simulink model "if_else"  (R2021a)
settings: Solver=VariableStepAuto  StartTime=0.0  StopTime=inf  MaxStep=0.01  RelTol=1e-3
libraries: simulink x1
settings Model: Creator=Aula  LastModifiedBy=Aula

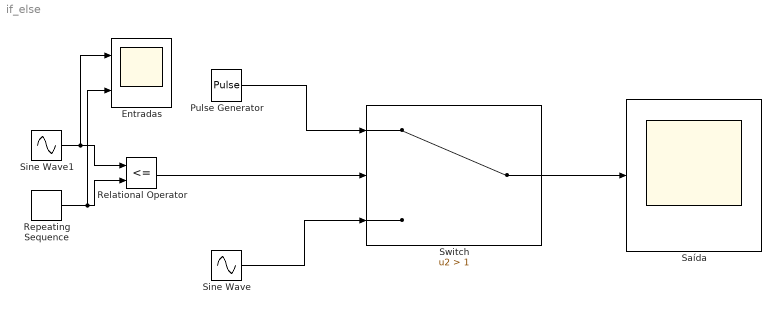
== system if_else ==
  Entradas : Scope  NumInputPorts=2
  Pulse Generator : DiscretePulseGenerator  PulseType=Time based  Period=5  PulseWidth=50
  Relational Operator : RelationalOperator  Operator=<=  OutDataTypeStr=boolean  RndMeth=Simplest
  Repeating Sequence : simulink/Sources/Repeating Sequence  rep_seq_t=[0 2]  rep_seq_y=[0 2]
  Saída : Scope
  Sine Wave : Sin  Amplitude=0.5  Frequency=5  SampleTime=0
  Sine Wave1 : Sin  Frequency=5  SampleTime=0
  Switch : Switch  Criteria=u2 > Threshold  Threshold=1
  wires:
  Sine Wave/1 -> Switch/3
  Pulse Generator/1 -> Switch/1
  Switch/1 -> Saída/1
  Relational Operator/1 -> Switch/2
  Sine Wave1/1 -> Entradas/1, Relational Operator/1
  Repeating Sequence/1 -> Relational Operator/2, Entradas/2
